simulink model "resp_of_closed_loop_buck_converter"  (R2016a)
settings: Solver=VariableStepAuto  StartTime=0.0  StopTime=1  RelTol=1e-3
libraries: simulink x1
settings Model: Creator=sourav mitra  LastModifiedBy=sourav mitra

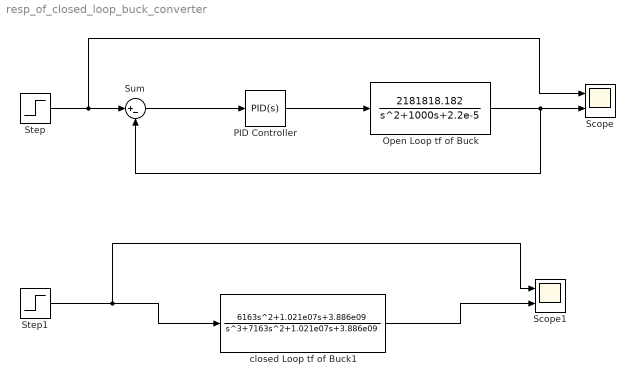
== system resp_of_closed_loop_buck_converter ==
  Open Loop tf of Buck : TransferFcn  Numerator=[2181818.182]  Denominator=[1 1000 2.2e-5]
  PID Controller : simulink/Continuous/PID Controller  Controller=PID  TimeDomain=Continuous-time  SampleTime=-1  IntegratorMethod=Forward Euler  FilterMethod=Forward Euler  Form=Parallel  UseFilter=on  ControllerParametersSource=internal  P=4.68108869404948  I=1781.09807280784  D=0.00282449827895437  N=710230.199325621  InitialConditionSource=internal  InitialConditionForIntegrator=0  InitialConditionForFilter=0  ExternalReset=none  LimitOutput=off  UpperSaturationLimit=inf  LowerSaturationLimit=-inf  LinearizeAsGain=on  AntiWindupMode=none  Kb=1  TrackingMode=off  Kt=1  PParamMin=[]  PParamMax=[]  IParamMin=[]  IParamMax=[]  DParamMin=[]  DParamMax=[]  NParamMin=[]  NParamMax=[]  KbParamMin=[]  KbParamMax=[]  KtParamMin=[]  KtParamMax=[]  POutMin=[]  POutMax=[]  IOutMin=[]  IOutMax=[]  DOutMin=[]  DOutMax=[]  NOutMin=[]  NOutMax=[]  KbOutMin=[]  KbOutMax=[]  KtOutMin=[]  KtOutMax=[]  IntegratorOutMin=[]  IntegratorOutMax=[]  FilterOutMin=[]  FilterOutMax=[]  SumOutMin=[]  SumOutMax=[]  SumI1OutMin=[]  SumI1OutMax=[]  SumI2OutMin=[]  SumI2OutMax=[]  SumI3OutMin=[]  SumI3OutMax=[]  SumDOutMin=[]  SumDOutMax=[]  SaturationOutMin=[]  SaturationOutMax=[]  IntegratorContinuousStateAttributes=''  IntegratorStateMustResolveToSignalObject=off  IntegratorRTWStateStorageClass=Auto  FilterContinuousStateAttributes=''  FilterStateMustResolveToSignalObject=off  FilterRTWStateStorageClass=Auto  DifferentiatorICPrevScaledInput=0  DifferentiatorOutMin=[]  DifferentiatorOutMax=[]
  Scope : Scope  NumInputPorts=2
  Scope1 : Scope  NumInputPorts=2
  Step : Step  Time=0.5  SampleTime=0
  Step1 : Step  Time=0.5  SampleTime=0
  Sum : Sum  Inputs=|+-
  closed Loop tf of Buck1 : TransferFcn  Numerator=[6163 1.021e07 3.886e09]  Denominator=[1 7163 1.021e07 3.886e09]
  wires:
  Step/1 -> Scope/1, Sum/1
  Sum/1 -> PID Controller/1
  PID Controller/1 -> Open Loop tf of Buck/1
  Open Loop tf of Buck/1 -> Sum/2, Scope/2
  Step1/1 -> closed Loop tf of Buck1/1, Scope1/1
  closed Loop tf of Buck1/1 -> Scope1/2
